simulink library "lib_controller"  (R2015a)
settings: Solver=ode45  StartTime=0.0  StopTime=10.0  RelTol=1e-3
values from neighbouring files (symbols this model uses):
  CG_0 = [0,0,0.02]'    [SetupComplete.m]
  g = 9.81    [SetupComplete.m]
  h_M = 0.064    [SetupComplete.m]
  I_BAC_0 = [ Ix,0,Ixz;0,Iy,0;Ixz,0,Iz]    [SetupComplete.m]
  l = 0.3450    (= 0.345)    [NDI_components.m]    (also in SetupComplete.m; robust_controller.m)
  m = 3.51    [SetupComplete.m]
  m_0 = 2.61    [SetupComplete.m]
  m_M = 0.300    (= 0.3)    [SetupComplete.m]
  T_sim = 0.01    [Run3Copter.m]
undefined symbols (not defined in the file or in its folder): Theta_1_roll_last, Theta_2_roll_last, Theta_3_roll_last, V_long_lastA_w_z, V_long_lastAoA, V_roll_last, V_yaw_last, W_long_lastA_w_z, W_long_lastAoA, W_roll_last, W_yaw_last
libraries: simulink x65, Adaptive_FaultTolerantControl x8, lib_controller x5, qcatlib x4, dspinverses x4, aerolibtransform2 x3, aerolib6dofsys x1
(part 9 of 10)

== matlab function lib_controller/Controller/NDI+CA Controller/4DOF NDI+CA Controller/F(X) ==
  data: fx output; prev_input input
function fx = fx(prev_input)
    % Calculates f_hat(x). The expression is calculated in NDI_components
    % x_dot = f(x) + g(x,u)
    %   g(x,u) ~= g(x,u0) + jac(g(x,u), u)(u0) * (u - u0)
    %   g(x,u) ~= h(x,u0) + jac(g(x,u), u)(u0) * u
    % x_dot = f_hat(x) + jac(g(x,u), u) * u
    %   f_hat(x) = f(x) + g(x,u0) - jac(g(x,u), u)(u0) *  u0
    %   g_hat(x) = jac(g(x,u), u)(u0)
    % x_dot = f_hat(x) + g_hat(x) * u
    Ixx = I_BAC(1,1);
    Iyy = I_BAC(2,2);
    Izz = I_BAC(3,3);
    Ixz = I_BAC(1,3);
    Iyz = I_BAC(2,3);
    cx = CG(1);
    cy = CG(2);
    cz = CG(3);
    tau1_0 = prev_input(1);
    eta1_0 = prev_input(2);
    gamma1_0 = prev_input(3);
    tau2_0 = prev_input(4);
    eta2_0 = prev_input(5);
    gamma2_0 = prev_input(6);
    tau3_0 = prev_input(7);
    eta3_0 = prev_input(8);
    gamma3_0 = prev_input(9);

    % TODO Precompute sines and cosines to improve performance. Some
    % repeated terms can also be precomputed
 fx = [...
               (88.941*(6.6073e-7*mass*P^2 + 0.000032054*mass*P*R - 6.6073e-7*mass*R^2 + 0.011243*V*mass*R + 0.011243*Gx - 0.011243*Q*W*mass - 5.7814e-6*eta1_0*mass*tau1_0*cos(eta1_0)))/mass;
 (88.941*(0.011243*Gy - 0.16865*eta1_0*tau1_0*cos(eta1_0) + 7.3537e-7*P*Q*mass + 0.00003163*Q*R*mass + 0.011243*P*W*mass - 0.011243*R*U*mass - 1.7153e-7*eta1_0*mass*tau1_0*sin(eta1_0)))/mass;
                                        -(88.941*(0.000016865*mass*P^2 + 0.011243*V*mass*P + 0.000016865*mass*Q^2 - 0.011243*U*mass*Q - 0.011243*Gz + 0.16865*eta1_0*tau1_0*sin(eta1_0)))/mass;
                                                                                                                               0.010171*eta1_0*tau1_0*sin(eta1_0) - 0.87546*Q*R - 0.043603*P*Q;
                                                                                                                  0.039177*P^2 + 0.90059*P*R - 0.039177*R^2 - 0.3428*eta1_0*tau1_0*cos(eta1_0);
                                                                                                                                0.043603*Q*R - 0.12686*P*Q - 0.20367*eta1_0*tau1_0*sin(eta1_0)];

== matlab function lib_controller/Controller/NDI+CA Controller/4DOF ANN+NDI+CA Controller - No massic update/Rotational Kinematics ==
  data: PQR output size=3; Eulerdot input size=3; Euler input size=3
function PQR = rot_kin(Eulerdot,Euler)
%solves rotational kinematic equations
Phi = Euler(1);
Theta = Euler(2);
Psi = Euler(3);
A = [1 sin(Phi)*tan(Theta) cos(Phi)*tan(Theta);
     0 cos(Phi) -sin(Phi);
     0 sin(Phi)*sec(Theta) cos(Phi)*sec(Theta)];
PQR = A'*Eulerdot;
end

== matlab function lib_controller/Controller/NDI+CA Controller/ 9DOF NDI+CA Controller - No massic update/F(X) 9DOF_UVWPQR ==
  data: fx output size=[6,1]; prev_input input size=[9,1]; gforce_body input size=[3,1]; omega_body input size=[3,1]; v_body input size=[3,1]
function fx = fx(prev_input, gforce_body, omega_body, v_body)
    % Calculates f_hat(x). The expression is calculated in NDI_components
    % x_dot = f(x) + g(x,u)
    %   g(x,u) ~= g(x,u0) + jac(g(x,u), u)(u0) * (u - u0)
    %   g(x,u) ~= h(x,u0) + jac(g(x,u), u)(u0) * u
    % x_dot = f_hat(x) + jac(g(x,u), u) * u
    %   f_hat(x) = f(x) + g(x,u0) - jac(g(x,u), u)(u0) *  u0
    %   g_hat(x) = jac(g(x,u), u)(u0)
    % x_dot = f_hat(x) + g_hat(x) * u
    tau1_0 = prev_input(1);
    eta1_0 = prev_input(2);
    gamma1_0 = prev_input(3);
    tau2_0 = prev_input(4);
    eta2_0 = prev_input(5);
    gamma2_0 = prev_input(6);
    tau3_0 = prev_input(7);
    eta3_0 = prev_input(8);
    gamma3_0 = prev_input(9);
    Gx =  gforce_body(1);
    Gy =  gforce_body(2);
    Gz =  gforce_body(3);
    U = v_body(1);
    V = v_body(2);
    W = v_body(3);
    P = omega_body(1);
    Q = omega_body(2);
    R = omega_body(3);

    % This matrix was precomputed in NDI_components.m
    % TODO Precompute sines and cosines to improve performance. Some
    % repeated terms can also be precomputed
    
 fx = [...
 5.88e-5*P^2 + 0.00285*P*R - 5.88e-5*R^2 + 1.0*V*R + 0.285*Gx - 1.0*Q*W + 4.27*gamma1_0*tau1_0*cos(gamma1_0) + 5.14e-4*gamma2_0*tau2_0*cos(gamma2_0) + 5.14e-4*gamma3_0*tau3_0*cos(gamma3_0) - 5.14e-4*eta1_0*tau1_0*cos(eta1_0)*cos(gamma1_0) + 4.27*eta2_0*tau2_0*cos(eta2_0)*cos(gamma2_0) + 4.27*eta3_0*tau3_0*cos(eta3_0)*cos(gamma3_0) + 0.038*eta1_0*tau1_0*cos(gamma1_0)*sin(eta1_0) - 0.019*eta2_0*tau2_0*cos(gamma2_0)*sin(eta2_0) - 0.019*eta3_0*tau3_0*cos(gamma3_0)*sin(eta3_0) + 0.038*gamma1_0*tau1_0*cos(eta1_0)*sin(gamma1_0) - 0.019*gamma2_0*tau2_0*cos(eta2_0)*sin(gamma2_0) - 0.019*gamma3_0*tau3_0*cos(eta3_0)*sin(gamma3_0) + 5.14e-4*gamma1_0*tau1_0*sin(eta1_0)*sin(gamma1_0) - 4.27*gamma2_0*tau2_0*sin(eta2_0)*sin(gamma2_0) - 4.27*gamma3_0*tau3_0*sin(eta3_0)*sin(gamma3_0);
        0.285*Gy + 6.54e-5*P*Q + 0.00281*Q*R + 1.0*P*W - 1.0*R*U - 6.56e-4*gamma1_0*tau1_0*cos(gamma1_0) - 4.27*gamma2_0*tau2_0*cos(gamma2_0) - 4.27*gamma3_0*tau3_0*cos(gamma3_0) - 4.27*eta1_0*tau1_0*cos(eta1_0)*cos(gamma1_0) - 3.21e-4*eta2_0*tau2_0*cos(eta2_0)*cos(gamma2_0) + 0.00163*eta3_0*tau3_0*cos(eta3_0)*cos(gamma3_0) - 1.53e-5*eta1_0*tau1_0*cos(gamma1_0)*sin(eta1_0) + 0.042*eta2_0*tau2_0*cos(gamma2_0)*sin(eta2_0) - 0.042*eta3_0*tau3_0*cos(gamma3_0)*sin(eta3_0) - 1.53e-5*gamma1_0*tau1_0*cos(eta1_0)*sin(gamma1_0) + 0.042*gamma2_0*tau2_0*cos(eta2_0)*sin(gamma2_0) - 0.042*gamma3_0*tau3_0*cos(eta3_0)*sin(gamma3_0) + 4.27*gamma1_0*tau1_0*sin(eta1_0)*sin(gamma1_0) + 3.21e-4*gamma2_0*tau2_0*sin(eta2_0)*sin(gamma2_0) - 0.00163*gamma3_0*tau3_0*sin(eta3_0)*sin(gamma3_0);
                                                                                                                                                                                                                                                                                                                                                                                                                                                - 0.0015*P^2 - 1.0*V*P - 0.0015*Q^2 + 1.0*U*Q + 0.285*Gz - 4.27*eta1_0*tau1_0*cos(gamma1_0)*sin(eta1_0) - 4.27*eta2_0*tau2_0*cos(gamma2_0)*sin(eta2_0) - 4.27*eta3_0*tau3_0*cos(gamma3_0)*sin(eta3_0) - 4.27*gamma1_0*tau1_0*cos(eta1_0)*sin(gamma1_0) - 4.27*gamma2_0*tau2_0*cos(eta2_0)*sin(gamma2_0) - 4.27*gamma3_0*tau3_0*cos(eta3_0)*sin(gamma3_0);
                                                        0.437*gamma1_0*tau1_0*cos(gamma1_0) - 0.876*Q*R - 0.0436*P*Q - 0.235*gamma2_0*tau2_0*cos(gamma2_0) - 0.235*gamma3_0*tau3_0*cos(gamma3_0) + 0.893*eta1_0*tau1_0*cos(eta1_0)*cos(gamma1_0) + 0.214*eta2_0*tau2_0*cos(eta2_0)*cos(gamma2_0) - 1.09*eta3_0*tau3_0*cos(eta3_0)*cos(gamma3_0) + 0.0102*eta1_0*tau1_0*cos(gamma1_0)*sin(eta1_0) - 28.0*eta2_0*tau2_0*cos(gamma2_0)*sin(eta2_0) + 28.0*eta3_0*tau3_0*cos(gamma3_0)*sin(eta3_0) + 0.0102*gamma1_0*tau1_0*cos(eta1_0)*sin(gamma1_0) - 28.0*gamma2_0*tau2_0*cos(eta2_0)*sin(gamma2_0) + 28.0*gamma3_0*tau3_0*cos(eta3_0)*sin(gamma3_0) - 0.893*gamma1_0*tau1_0*sin(eta1_0)*sin(gamma1_0) - 0.214*gamma2_0*tau2_0*sin(eta2_0)*sin(gamma2_0) + 1.09*gamma3_0*tau3_0*sin(eta3_0)*sin(gamma3_0);
                                                  0.0392*P^2 + 0.901*P*R - 0.0392*R^2 + 0.11*gamma1_0*tau1_0*cos(gamma1_0) + 0.343*gamma2_0*tau2_0*cos(gamma2_0) + 0.343*gamma3_0*tau3_0*cos(gamma3_0) - 0.343*eta1_0*tau1_0*cos(eta1_0)*cos(gamma1_0) + 0.11*eta2_0*tau2_0*cos(eta2_0)*cos(gamma2_0) + 0.11*eta3_0*tau3_0*cos(eta3_0)*cos(gamma3_0) + 25.3*eta1_0*tau1_0*cos(gamma1_0)*sin(eta1_0) - 12.7*eta2_0*tau2_0*cos(gamma2_0)*sin(eta2_0) - 12.7*eta3_0*tau3_0*cos(gamma3_0)*sin(eta3_0) + 25.3*gamma1_0*tau1_0*cos(eta1_0)*sin(gamma1_0) - 12.7*gamma2_0*tau2_0*cos(eta2_0)*sin(gamma2_0) - 12.7*gamma3_0*tau3_0*cos(eta3_0)*sin(gamma3_0) + 0.343*gamma1_0*tau1_0*sin(eta1_0)*sin(gamma1_0) - 0.11*gamma2_0*tau2_0*sin(eta2_0)*sin(gamma2_0) - 0.11*gamma3_0*tau3_0*sin(eta3_0)*sin(gamma3_0);
                                                           0.0436*Q*R - 0.127*P*Q - 0.0102*gamma1_0*tau1_0*cos(gamma1_0) + 7.53*gamma2_0*tau2_0*cos(gamma2_0) + 7.53*gamma3_0*tau3_0*cos(gamma3_0) - 15.1*eta1_0*tau1_0*cos(eta1_0)*cos(gamma1_0) - 13.0*eta2_0*tau2_0*cos(eta2_0)*cos(gamma2_0) + 13.0*eta3_0*tau3_0*cos(eta3_0)*cos(gamma3_0) - 0.204*eta1_0*tau1_0*cos(gamma1_0)*sin(eta1_0) + 0.855*eta2_0*tau2_0*cos(gamma2_0)*sin(eta2_0) - 0.448*eta3_0*tau3_0*cos(gamma3_0)*sin(eta3_0) - 0.204*gamma1_0*tau1_0*cos(eta1_0)*sin(gamma1_0) + 0.855*gamma2_0*tau2_0*cos(eta2_0)*sin(gamma2_0) - 0.448*gamma3_0*tau3_0*cos(eta3_0)*sin(gamma3_0) + 15.1*gamma1_0*tau1_0*sin(eta1_0)*sin(gamma1_0) + 13.0*gamma2_0*tau2_0*sin(eta2_0)*sin(gamma2_0) - 13.0*gamma3_0*tau3_0*sin(eta3_0)*sin(gamma3_0)];

== matlab function lib_controller/Controller/NDI+CA Controller/ 9DOF NDI+CA Controller - No massic update/G(X) 9DOF_UVWPQR ==
  data: gx output size=[6,9]; prev_input input size=[9,1]
function gx = gx(prev_input)
    % Calculates f_hat(x). The expression is calculated in NDI_components
    % x_dot = f(x) + g(x,u)
    %   g(x,u) ~= g(x,u0) + jac(g(x,u), u)(u0) * (u - u0)
    %   g(x,u) ~= h(x,u0) + jac(g(x,u), u)(u0) * u
    % x_dot = f_hat(x) + jac(g(x,u), u) * u
    %   f_hat(x) = f(x) + g(x,u0) - jac(g(x,u), u)(u0) *  u0
    %   g_hat(x) = jac(g(x,u), u)(u0)
    % x_dot = f_hat(x) + g_hat(x) * u
    tau1_0 = prev_input(1);
    eta1_0 = prev_input(2);
    gamma1_0 = prev_input(3);
    tau2_0 = prev_input(4);
    eta2_0 = prev_input(5);
    gamma2_0 = prev_input(6);
    tau3_0 = prev_input(7);
    eta3_0 = prev_input(8);
    gamma3_0 = prev_input(9);
    
    % This matrix was precomputed in NDI_components.m
    % TODO Precompute sines and cosines to improve performance. Some
    % repeated terms can also be precomputed
    gx = [...
   5.14e-4*cos(gamma1_0)*sin(eta1_0) - 4.27*sin(gamma1_0) + 0.038*cos(eta1_0)*cos(gamma1_0),  5.14e-4*tau1_0*cos(eta1_0)*cos(gamma1_0) - 0.038*tau1_0*cos(gamma1_0)*sin(eta1_0), - 4.27*tau1_0*cos(gamma1_0) - 0.038*tau1_0*cos(eta1_0)*sin(gamma1_0) - 5.14e-4*tau1_0*sin(eta1_0)*sin(gamma1_0), - 5.14e-4*sin(gamma2_0) - 4.27*cos(gamma2_0)*sin(eta2_0) - 0.019*cos(eta2_0)*cos(gamma2_0),    0.019*tau2_0*cos(gamma2_0)*sin(eta2_0) - 4.27*tau2_0*cos(eta2_0)*cos(gamma2_0), 0.019*tau2_0*cos(eta2_0)*sin(gamma2_0) - 5.14e-4*tau2_0*cos(gamma2_0) + 4.27*tau2_0*sin(eta2_0)*sin(gamma2_0), - 5.14e-4*sin(gamma3_0) - 4.27*cos(gamma3_0)*sin(eta3_0) - 0.019*cos(eta3_0)*cos(gamma3_0),    0.019*tau3_0*cos(gamma3_0)*sin(eta3_0) - 4.27*tau3_0*cos(eta3_0)*cos(gamma3_0), 0.019*tau3_0*cos(eta3_0)*sin(gamma3_0) - 5.14e-4*tau3_0*cos(gamma3_0) + 4.27*tau3_0*sin(eta3_0)*sin(gamma3_0);
 6.56e-4*sin(gamma1_0) + 4.27*cos(gamma1_0)*sin(eta1_0) - 1.53e-5*cos(eta1_0)*cos(gamma1_0),   4.27*tau1_0*cos(eta1_0)*cos(gamma1_0) + 1.53e-5*tau1_0*cos(gamma1_0)*sin(eta1_0), 6.56e-4*tau1_0*cos(gamma1_0) + 1.53e-5*tau1_0*cos(eta1_0)*sin(gamma1_0) - 4.27*tau1_0*sin(eta1_0)*sin(gamma1_0),   4.27*sin(gamma2_0) + 3.21e-4*cos(gamma2_0)*sin(eta2_0) + 0.042*cos(eta2_0)*cos(gamma2_0), 3.21e-4*tau2_0*cos(eta2_0)*cos(gamma2_0) - 0.042*tau2_0*cos(gamma2_0)*sin(eta2_0), 4.27*tau2_0*cos(gamma2_0) - 0.042*tau2_0*cos(eta2_0)*sin(gamma2_0) - 3.21e-4*tau2_0*sin(eta2_0)*sin(gamma2_0),   4.27*sin(gamma3_0) - 0.00163*cos(gamma3_0)*sin(eta3_0) - 0.042*cos(eta3_0)*cos(gamma3_0), 0.042*tau3_0*cos(gamma3_0)*sin(eta3_0) - 0.00163*tau3_0*cos(eta3_0)*cos(gamma3_0), 4.27*tau3_0*cos(gamma3_0) + 0.042*tau3_0*cos(eta3_0)*sin(gamma3_0) + 0.00163*tau3_0*sin(eta3_0)*sin(gamma3_0);
                                                            -4.27*cos(eta1_0)*cos(gamma1_0),                                              4.27*tau1_0*cos(gamma1_0)*sin(eta1_0),                                                                           4.27*tau1_0*cos(eta1_0)*sin(gamma1_0),                                                            -4.27*cos(eta2_0)*cos(gamma2_0),                                             4.27*tau2_0*cos(gamma2_0)*sin(eta2_0),                                                                         4.27*tau2_0*cos(eta2_0)*sin(gamma2_0),                                                            -4.27*cos(eta3_0)*cos(gamma3_0),                                             4.27*tau3_0*cos(gamma3_0)*sin(eta3_0),                                                                         4.27*tau3_0*cos(eta3_0)*sin(gamma3_0);
   0.0102*cos(eta1_0)*cos(gamma1_0) - 0.893*cos(gamma1_0)*sin(eta1_0) - 0.437*sin(gamma1_0), - 0.893*tau1_0*cos(eta1_0)*cos(gamma1_0) - 0.0102*tau1_0*cos(gamma1_0)*sin(eta1_0),   0.893*tau1_0*sin(eta1_0)*sin(gamma1_0) - 0.0102*tau1_0*cos(eta1_0)*sin(gamma1_0) - 0.437*tau1_0*cos(gamma1_0),     0.235*sin(gamma2_0) - 0.214*cos(gamma2_0)*sin(eta2_0) - 28.0*cos(eta2_0)*cos(gamma2_0),    28.0*tau2_0*cos(gamma2_0)*sin(eta2_0) - 0.214*tau2_0*cos(eta2_0)*cos(gamma2_0),   0.235*tau2_0*cos(gamma2_0) + 28.0*tau2_0*cos(eta2_0)*sin(gamma2_0) + 0.214*tau2_0*sin(eta2_0)*sin(gamma2_0),      0.235*sin(gamma3_0) + 1.09*cos(gamma3_0)*sin(eta3_0) + 28.0*cos(eta3_0)*cos(gamma3_0),     1.09*tau3_0*cos(eta3_0)*cos(gamma3_0) - 28.0*tau3_0*cos(gamma3_0)*sin(eta3_0),    0.235*tau3_0*cos(gamma3_0) - 28.0*tau3_0*cos(eta3_0)*sin(gamma3_0) - 1.09*tau3_0*sin(eta3_0)*sin(gamma3_0);
      0.343*cos(gamma1_0)*sin(eta1_0) - 0.11*sin(gamma1_0) + 25.3*cos(eta1_0)*cos(gamma1_0),     0.343*tau1_0*cos(eta1_0)*cos(gamma1_0) - 25.3*tau1_0*cos(gamma1_0)*sin(eta1_0),    - 0.11*tau1_0*cos(gamma1_0) - 25.3*tau1_0*cos(eta1_0)*sin(gamma1_0) - 0.343*tau1_0*sin(eta1_0)*sin(gamma1_0),    - 0.343*sin(gamma2_0) - 0.11*cos(gamma2_0)*sin(eta2_0) - 12.7*cos(eta2_0)*cos(gamma2_0),     12.7*tau2_0*cos(gamma2_0)*sin(eta2_0) - 0.11*tau2_0*cos(eta2_0)*cos(gamma2_0),    12.7*tau2_0*cos(eta2_0)*sin(gamma2_0) - 0.343*tau2_0*cos(gamma2_0) + 0.11*tau2_0*sin(eta2_0)*sin(gamma2_0),    - 0.343*sin(gamma3_0) - 0.11*cos(gamma3_0)*sin(eta3_0) - 12.7*cos(eta3_0)*cos(gamma3_0),     12.7*tau3_0*cos(gamma3_0)*sin(eta3_0) - 0.11*tau3_0*cos(eta3_0)*cos(gamma3_0),    12.7*tau3_0*cos(eta3_0)*sin(gamma3_0) - 0.343*tau3_0*cos(gamma3_0) + 0.11*tau3_0*sin(eta3_0)*sin(gamma3_0);
    0.0102*sin(gamma1_0) + 15.1*cos(gamma1_0)*sin(eta1_0) - 0.204*cos(eta1_0)*cos(gamma1_0),     15.1*tau1_0*cos(eta1_0)*cos(gamma1_0) + 0.204*tau1_0*cos(gamma1_0)*sin(eta1_0),    0.0102*tau1_0*cos(gamma1_0) + 0.204*tau1_0*cos(eta1_0)*sin(gamma1_0) - 15.1*tau1_0*sin(eta1_0)*sin(gamma1_0),      13.0*cos(gamma2_0)*sin(eta2_0) - 7.53*sin(gamma2_0) + 0.855*cos(eta2_0)*cos(gamma2_0),    13.0*tau2_0*cos(eta2_0)*cos(gamma2_0) - 0.855*tau2_0*cos(gamma2_0)*sin(eta2_0),  - 7.53*tau2_0*cos(gamma2_0) - 0.855*tau2_0*cos(eta2_0)*sin(gamma2_0) - 13.0*tau2_0*sin(eta2_0)*sin(gamma2_0),    - 7.53*sin(gamma3_0) - 13.0*cos(gamma3_0)*sin(eta3_0) - 0.448*cos(eta3_0)*cos(gamma3_0),    0.448*tau3_0*cos(gamma3_0)*sin(eta3_0) - 13.0*tau3_0*cos(eta3_0)*cos(gamma3_0),    0.448*tau3_0*cos(eta3_0)*sin(gamma3_0) - 7.53*tau3_0*cos(gamma3_0) + 13.0*tau3_0*sin(eta3_0)*sin(gamma3_0)];
 
    
    
    
    
%  0.038016*cos(eta1_0) + 0.00051422*sin(eta1_0), 0.00051422*tau1_0*cos(eta1_0) - 0.038016*tau1_0*sin(eta1_0),    -4.2737*tau1_0, -0.019008,    -4.2737*tau2_0, -0.00051422*tau2_0, -0.019008,   -4.2737*tau3_0, -0.00051422*tau3_0;
%   4.2748*sin(eta1_0) - 0.000015257*cos(eta1_0),  4.2748*tau1_0*cos(eta1_0) + 0.000015257*tau1_0*sin(eta1_0), 0.00065622*tau1_0,  0.042029, 0.00032056*tau2_0,      4.2732*tau2_0, -0.041999, -0.001633*tau3_0,      4.2732*tau3_0;
%                            -4.2735*cos(eta1_0),                                   4.2735*tau1_0*sin(eta1_0),                 0,   -4.2735,                 0,                  0,   -4.2735,                0,                  0;
%     0.010171*cos(eta1_0) - 0.89255*sin(eta1_0),  - 0.89255*tau1_0*cos(eta1_0) - 0.010171*tau1_0*sin(eta1_0),   -0.43748*tau1_0,    -28.02,   -0.21371*tau2_0,     0.23535*tau2_0,    27.999,    1.0887*tau3_0,     0.23535*tau3_0;
%       25.344*cos(eta1_0) + 0.34281*sin(eta1_0),      0.34281*tau1_0*cos(eta1_0) - 25.344*tau1_0*sin(eta1_0),   -0.11019*tau1_0,   -12.672,   -0.11019*tau2_0,    -0.34281*tau2_0,   -12.672,  -0.11019*tau3_0,    -0.34281*tau3_0;
%        15.06*sin(eta1_0) - 0.20367*cos(eta1_0),       15.06*tau1_0*cos(eta1_0) + 0.20367*tau1_0*sin(eta1_0),   0.010171*tau1_0,   0.85486,     13.029*tau2_0,     -7.5251*tau2_0,  -0.44753,    -13.05*tau3_0,     -7.5251*tau3_0];

== matlab function lib_controller/Controller/NDI+CA Controller/4DOF ANN+NDI+CA Controller - No massic update/G(X) 4DOF_WPQR ==
  data: gx output size=[4,4]; prev_input input size=[9,1]
function gx = gx(prev_input)
    % Calculates f_hat(x). The expression is calculated in NDI_components
    % x_dot = f(x) + g(x,u)
    %   g(x,u) ~= g(x,u0) + jac(g(x,u), u)(u0) * (u - u0)
    %   g(x,u) ~= h(x,u0) + jac(g(x,u), u)(u0) * u
    % x_dot = f_hat(x) + jac(g(x,u), u) * u
    %   f_hat(x) = f(x) + g(x,u0) - jac(g(x,u), u)(u0) *  u0
    %   g_hat(x) = jac(g(x,u), u)(u0)
    % x_dot = f_hat(x) + g_hat(x) * u
    tau1_0 = prev_input(1);
    eta1_0 = prev_input(2);
    gamma1_0 = prev_input(3);
    tau2_0 = prev_input(4);
    eta2_0 = prev_input(5);
    gamma2_0 = prev_input(6);
    tau3_0 = prev_input(7);
    eta3_0 = prev_input(8);
    gamma3_0 = prev_input(9);
    
    % This matrix was precomputed in NDI_components.m
    % TODO Precompute sines and cosines to improve performance. Some
    % repeated terms can also be precomputed
    
    % Kt = 29.6 Kq = 0.3
    gx = [...
                          -7.379*cos(eta1_0),                                7.379*tau1_0*sin(eta1_0), -7.379,  -7.379;
     0.04359*cos(eta1_0) - 1.541*sin(eta1_0), - 1.541*tau1_0*cos(eta1_0) - 0.04359*tau1_0*sin(eta1_0), -48.41,   48.32;
       43.76*cos(eta1_0) + 1.469*sin(eta1_0),     1.469*tau1_0*cos(eta1_0) - 43.76*tau1_0*sin(eta1_0), -21.88,  -21.88;
       26.0*sin(eta1_0) - 0.8729*cos(eta1_0),     26.0*tau1_0*cos(eta1_0) + 0.8729*tau1_0*sin(eta1_0),  1.997, -0.2515];
 
% Kt = 15 Kq = 0.07
%                        -4.274*cos(eta1_0),                                 4.274*tau1_0*sin(eta1_0), -4.274,  -4.274;
%  0.01017*cos(eta1_0) - 0.8926*sin(eta1_0), - 0.8926*tau1_0*cos(eta1_0) - 0.01017*tau1_0*sin(eta1_0), -28.02,    28.0;
%    25.34*cos(eta1_0) + 0.3428*sin(eta1_0),     0.3428*tau1_0*cos(eta1_0) - 25.34*tau1_0*sin(eta1_0), -12.67,  -12.67;
%    15.06*sin(eta1_0) - 0.2037*cos(eta1_0),     15.06*tau1_0*cos(eta1_0) + 0.2037*tau1_0*sin(eta1_0), 0.8549, -0.4475];

== matlab function lib_controller/Controller/NDI+CA Controller/4DOF ANN+NDI+CA Controller - No massic update/Adaptive NN/Crossed NN/Cross NN ==
  data: X_bar input size=[30,1]; v_ad_comp output size=4; e input size=6; P input size=[6,6]; B input size=[6,4]; learning_rate input size=1; Reg_param input size=2; W input size=[4,51]; V input size=[50,30]; v_ad output size=4; Z_norm_unit output size=1; T_sim parameter size=1; W_update output size=[4,51]; V_update output size=[50,30]
function [v_ad_comp,v_ad,Z_norm_unit,W_update,V_update]  = Cross_NN(X_bar,e, P, B,learning_rate,Reg_param,W,V,T_sim)

%% Compute prelimiary parameters 
zeta= e'*P*B;

%% Feedforward
z = V*X_bar;
s=sigmoid(V*X_bar);

sigma = [1 ; s ];
% v_ad = W*sigma;

sigma_grad = (sigma.*(ones(size(sigma))-sigma));

%% Compute the gradients or adaptation laws
Gamma_w= learning_rate; % W learnign rate
Gamma_v= learning_rate; %V learning rate
lambda_v = Reg_param(1);
lambda_w = Reg_param(2);

V_dot=zeros(size(V));
W_dot=zeros(size(W));

W_dot= -Gamma_w*(  (sigma - sigma_grad.*[1;z] )*zeta  )';
W_dot(:,2:end)= W_dot(:,2:end) - Gamma_w*lambda_w*norm(zeta)*(W(:,2:end));

M = W'*zeta'.*sigma_grad ;
V_dot= -Gamma_v*( M(2:end)*X_bar'  );
V_dot(:,2:end)= V_dot(:,2:end) - Gamma_v*lambda_v*norm(zeta).*V(:,2:end);

% % % % Other way: Based on notes of Andrew NG
% % % 
% % % delta2=W'*zeta'.*sigma_grad;
% % % 
% % % V_dot = - Gamma_v*( delta2(2:end)*X_bar');
% % % V_dot(:,2:end)= V_dot(:,2:end) - Gamma_v*lambda*norm(zeta).*V(:,2:end);
% % % 
% % % W_dot = - Gamma_w*( sigma*zeta)';
% % % W_dot(:,2:end)= W_dot(:,2:end) - Gamma_w*lambda*norm(zeta)*(W(:,2:end));

%% Adaptation scalled with loop time
W_update = W + T_sim*W_dot;
V_update = V + T_sim*V_dot;

%% Re-compute v_ad
s=sigmoid(V_update*X_bar);

sigma = [1 ; s(:,1) ];
v_ad = W_update*sigma;

%% Compute v_ad_comp (add robustifying terms)
Z = [ V,zeros(size(V,1),size(W,2));
    zeros(size(W,1),size(V,2)),W];
    
Z_norm = norm(Z,'fro');
% Z_max = 2*min(size(W,1),size(W,2) )*min(size(V,1),size(V,2));
Z_max = 1;
Z_norm_unit = Z_norm;

% K_r0= 0.02;
% K_r1= 0;
K_r0= 1;
K_r1= 1;

v_r0 = -K_r0*zeta';
v_r1 = -K_r1*(Z_norm+Z_max)*zeta';

v_ad_comp = v_ad + v_r1 +v_r0;
end

== matlab function lib_controller/Controller/NDI+CA Controller/4DOF ANN+NDI+CA Controller - No massic update/Rotational Kinematics1 ==
  data: PQR input size=3; Eulerdot output size=3; Euler input size=3
function Eulerdot = rot_kin(PQR,Euler)
%solves rotational kinematic equations
Phi = Euler(1);
Theta = Euler(2);
Psi = Euler(3);
A = [1 sin(Phi)*tan(Theta) cos(Phi)*tan(Theta);
     0 cos(Phi) -sin(Phi);
     0 sin(Phi)*sec(Theta) cos(Phi)*sec(Theta)];
Eulerdot = A*PQR;
end

== matlab function lib_controller/Controller/NDI+CA Controller/4DOF ANN+NDI+CA Controller - No massic update/Sigmoid /MATLAB Function ==
  data: u input; y output; a input
function y = sigmoid_a(u,a)

y = 2.0 ./ (1.0 + exp(-a*u(:)))-1;

== matlab function lib_controller/Controller/NDI+CA Controller/4DOF ANN+NDI+CA Controller - No massic update/F(X) ==
  data: fx output size=[4,1]; prev_input input size=[9,1]; gforce_body input size=[3,1]; omega_body input size=[3,1]; v_body input size=[3,1]
function fx = fx(prev_input, gforce_body, omega_body, v_body)
    % Calculates f_hat(x). The expression is calculated in NDI_components
    % x_dot = f(x) + g(x,u)
    %   g(x,u) ~= g(x,u0) + jac(g(x,u), u)(u0) * (u - u0)
    %   g(x,u) ~= h(x,u0) + jac(g(x,u), u)(u0) * u
    % x_dot = f_hat(x) + jac(g(x,u), u) * u
    %   f_hat(x) = f(x) + g(x,u0) - jac(g(x,u), u)(u0) *  u0
    %   g_hat(x) = jac(g(x,u), u)(u0)
    % x_dot = f_hat(x) + g_hat(x) * u
    tau1_0 = prev_input(1);
    eta1_0 = prev_input(2);
    gamma1_0 = prev_input(3);
    tau2_0 = prev_input(4);
    eta2_0 = prev_input(5);
    gamma2_0 = prev_input(6);
    tau3_0 = prev_input(7);
    eta3_0 = prev_input(8);
    gamma3_0 = prev_input(9);
    Gx =  gforce_body(1);
    Gy =  gforce_body(2);
    Gz =  gforce_body(3);
    U = v_body(1);
    V = v_body(2);
    W = v_body(3);
    P = omega_body(1);
    Q = omega_body(2);
    R = omega_body(3);

    % This matrix was precomputed in NDI_components.m
    % TODO Precompute sines and cosines to improve performance. Some
    % repeated terms can also be precomputed
    
 % Kt = 29.6 Kq = 0.3
 fx = [... 
                    - 0.0015*P^2 - 1.0*V*P - 0.0015*Q^2 + U*Q + 0.2849*Gz - 7.379*eta1_0*tau1_0*sin(eta1_0);
              1.541*eta1_0*tau1_0*cos(eta1_0) - 0.8756*Q*R - 0.0436*P*Q + 0.04359*eta1_0*tau1_0*sin(eta1_0);
 0.03918*P^2 + 0.9007*P*R - 0.03918*R^2 - 1.469*eta1_0*tau1_0*cos(eta1_0) + 43.76*eta1_0*tau1_0*sin(eta1_0);
                0.0436*Q*R - 0.1269*P*Q - 26.0*eta1_0*tau1_0*cos(eta1_0) - 0.8729*eta1_0*tau1_0*sin(eta1_0)];    
 
% Kt = 15 Kq = 0.07
%                          - 0.0015*P^2 - 1.0*V*P - 0.0015*Q^2 + 1.0*U*Q + 0.2849*Gz - 4.2735*eta1_0*tau1_0*sin(eta1_0);
%                   0.89255*eta1_0*tau1_0*cos(eta1_0) - 0.87555*Q*R - 0.043605*P*Q + 0.010171*eta1_0*tau1_0*sin(eta1_0);
%      0.039179*P^2 + 0.90066*P*R - 0.039179*R^2 - 0.34281*eta1_0*tau1_0*cos(eta1_0) + 25.344*eta1_0*tau1_0*sin(eta1_0);
%                      0.043605*Q*R - 0.12686*P*Q - 15.06*eta1_0*tau1_0*cos(eta1_0) - 0.20367*eta1_0*tau1_0*sin(eta1_0)];

== matlab function lib_controller/Controller/NDI+CA Controller/4DOF ANN+NDI+CA Controller - No massic update/Rotational Kinematics2 ==
  data: PQR output size=3; Eulerdot input size=3; Euler input size=3
function PQR = rot_kin(Eulerdot,Euler)
%solves rotational kinematic equations
Phi = Euler(1);
Theta = Euler(2);
Psi = Euler(3);
A = [1 sin(Phi)*tan(Theta) cos(Phi)*tan(Theta);
     0 cos(Phi) -sin(Phi);
     0 sin(Phi)*sec(Theta) cos(Phi)*sec(Theta)];
PQR = A'*Eulerdot;
end

== matlab function lib_controller/Controller/NDI+CA Controller/4DOF ANN+NDI+CA Controller - No massic update/On-line (adaptive) multi-layer NNs/Pitch Channel/Long HL NN A_w_z/Long NN ==
  data: X_bar input size=[10,1]; v_ad_comp output; e input; F input; Ks input; B input; Long_learnign_rate input size=1; Long_reg_param input size=1; W input size=[1,31]; V input size=[30,10]; v_ad output; Z_norm_unit output; T_sim parameter; W_update output; V_update output
function [v_ad_comp,v_ad,Z_norm_unit,W_update,V_update]  = Long_AoA_NN(X_bar,e, F, Ks,B,Long_learnign_rate,Long_reg_param,W,V,T_sim)

%% Compute prelimiary parametes Ks(1)=K_b_alpha  and Ks(2) = K_b_q
P = [   1/Ks(1) , F/(Ks(1)^2+Ks(1)*Ks(2));
     1/(Ks(1)^2+Ks(1)*Ks(2)) ,(Ks(1)^2+Ks(1)*Ks(2)+F^2)/(Ks(2)^2*Ks(1)+Ks(2)*Ks(1)^2) ];
zeta= e'*P*B;
s=zeros(30,1);
z=s;
%% Feedforward
z = V*X_bar;
s=sigmoid(V*X_bar);

sigma = [1 ; s ];
% v_ad = W*sigma;

sigma_grad = (sigma.*(ones(size(sigma))-sigma));

%% Compute the gradients or adaptation laws
Gamma_w= Long_learnign_rate; % W learnign rate
Gamma_v= Long_learnign_rate; %V learning rate
lambda = Long_reg_param;

V_dot=zeros(size(V));
W_dot=zeros(size(W'));

W_dot= -Gamma_w*(  (sigma - sigma_grad.*[1;z] ).*zeta  );
W_dot(2:end,1)= W_dot(2:end,1) - Gamma_w*lambda*norm(zeta)*(W(:,2:end))';

M = W'*zeta.*sigma_grad ;
V_dot= -Gamma_v*( M(2:end)*X_bar'  );
V_dot(:,2:end)= V_dot(:,2:end) - Gamma_v*lambda*norm(zeta).*V(:,2:end);


% % % Other way: Based on notes of Andrew NG
% % W_dot=zeros(size(W));
% % delta2=W'*zeta.*sigma_grad;
% % 
% % V_dot = - Gamma_v*( delta2(2:end)*X_bar');
% % V_dot(:,2:end)= V_dot(:,2:end) - Gamma_v*lambda*norm(zeta).*V(:,2:end);
% % 
% % W_dot = - Gamma_w*( zeta*sigma');
% % W_dot(:,2:end)= W_dot(:,2:end) - Gamma_w*lambda*norm(zeta)*(W(:,2:end));
% % 
% % W_dot = W_dot';


%% Adaptation
W_update = W + T_sim*W_dot';
V_update = V + T_sim*V_dot;

%% re-compute v_ad

z = V*X_bar;
s=sigmoid(V*X_bar);

sigma = [1 ; s(:,1) ];
v_ad = W*sigma;

%% Compute v_ad_comp
Z = [ V,zeros(size(V,1),size(W,2));
    zeros(size(W,1),size(V,2)),W];
    
Z_norm = norm(Z,'fro');
Z_max = 2*min(size(W,1),size(W,2) )*min( size(V,1),size(V,2) );
Z_norm_unit = Z_norm/Z_max;

K_r0= 0.1;
K_r1= 0.001;
v_r0 = -K_r0*zeta;
v_r1 = -K_r1*(Z_norm+Z_max)*zeta;

v_ad_comp = v_ad + v_r1 +v_r0;


end

== matlab function lib_controller/Controller/NDI+CA Controller/4DOF ANN+NDI+CA Controller - No massic update/On-line (adaptive) multi-layer NNs/Pitch Channel/Long HL NN AoA/Long NN ==
  data: X_bar input size=[10,1]; v_ad_comp output; e input; Ks input; B input; Long_learnign_rate input size=1; Long_reg_param input size=1; W input size=[1,31]; V input size=[30,10]; v_ad output; Z_norm_unit output; T_sim parameter; W_update output; V_update output
function [v_ad_comp,v_ad,Z_norm_unit,W_update,V_update]  = Long_AoA_NN(X_bar,e, Ks,B,Long_learnign_rate,Long_reg_param,W,V,T_sim)

%% Compute prelimiary parametes Ks(1)=K_b_alpha  and Ks(2) = K_b_q
P = [   1/Ks(1) , 1/(Ks(1)^2+Ks(1)*Ks(2));
     1/(Ks(1)^2+Ks(1)*Ks(2)) ,(Ks(1)^2+Ks(1)*Ks(2)+1)/(Ks(2)^2*Ks(1)+Ks(2)*Ks(1)^2) ];
zeta= e'*P*B;
s=zeros(30,1);
z=s;
%% Feedforward
z = V*X_bar;
s=sigmoid(V*X_bar);

sigma = [1 ; s ];
% v_ad = W*sigma;

sigma_grad = (sigma.*(ones(size(sigma))-sigma));

%% Compute the gradients or adaptation laws
Gamma_w= Long_learnign_rate; % W learnign rate
Gamma_v= Long_learnign_rate; %V learning rate
lambda = Long_reg_param;

V_dot=zeros(size(V));
W_dot=zeros(size(W'));

W_dot= -Gamma_w*(  (sigma - sigma_grad.*[1;z] ).*zeta  );
W_dot(2:end,1)= W_dot(2:end,1) - Gamma_w*lambda*norm(zeta)*(W(:,2:end))';

M = W'*zeta.*sigma_grad ;
V_dot= -Gamma_v*( M(2:end)*X_bar'  );
V_dot(:,2:end)= V_dot(:,2:end) - Gamma_v*lambda*norm(zeta).*V(:,2:end);


% % % Other way: Based on notes of Andrew NG
% % W_dot=zeros(size(W));
% % delta2=W'*zeta.*sigma_grad;
% % 
% % V_dot = - Gamma_v*( delta2(2:end)*X_bar');
% % V_dot(:,2:end)= V_dot(:,2:end) - Gamma_v*lambda*norm(zeta).*V(:,2:end);
% % 
% % W_dot = - Gamma_w*( zeta*sigma');
% % W_dot(:,2:end)= W_dot(:,2:end) - Gamma_w*lambda*norm(zeta)*(W(:,2:end));
% % 
% % W_dot = W_dot';


%% Adaptation
W_update = W + T_sim*W_dot';
V_update = V + T_sim*V_dot;

%% re-compute v_ad

z = V*X_bar;
s=sigmoid(V*X_bar);

sigma = [1 ; s(:,1) ];
v_ad = W*sigma;

%% Compute v_ad_comp
Z = [ V,zeros(size(V,1),size(W,2));
    zeros(size(W,1),size(V,2)),W];
    
Z_norm = norm(Z,'fro');
Z_max = 2*min(size(W,1),size(W,2) )*min( size(V,1),size(V,2) );
Z_norm_unit = Z_norm;

K_r0= 0.02;
K_r1= 0;
v_r0 = -K_r0*zeta;
v_r1 = -K_r1*(Z_norm+Z_max)*zeta;

v_ad_comp = v_ad + v_r1 +v_r0;


end

== matlab function lib_controller/Controller/NDI+CA Controller/4DOF ANN+NDI+CA Controller - No massic update/On-line (adaptive) multi-layer NNs/Roll Channel/Roll 1HL NN/Roll NN ==
  data: X_bar input size=[12,1]; v_ad_comp output; e input; P input; B input; Roll_learnign_rate input size=1; Roll_reg_param input size=1; W input size=[1,31]; V input size=[30,12]; v_ad output; Z_norm_unit output; T_sim parameter; W_update output size=[1,31]; V_update output size=[30,12]
function [v_ad_comp,v_ad,Z_norm_unit,W_update,V_update]  = Roll_NN(X_bar,e,P,B,Roll_learnign_rate,Roll_reg_param,W,V,T_sim)

%% Compute prelimiary parametes
zeta= e'*P*B;
s=zeros(30,1);
z=s;
%% Feedforward
z = V*X_bar;
s=sigmoid(V*X_bar);

sigma = [1 ; s ];
% v_ad = W*sigma;

sigma_grad = (sigma.*(ones(size(sigma))-sigma));

%% Compute the gradients or adaptation laws
Gamma_w= Roll_learnign_rate; % W learnign rate
Gamma_v= Roll_learnign_rate; %V learning rate
lambda = Roll_reg_param;

V_dot=zeros(size(V));
W_dot=zeros(size(W'));

W_dot= -Gamma_w*(  (sigma - sigma_grad.*[1;z] ).*zeta  );
W_dot(2:end,1)= W_dot(2:end,1) - Gamma_w*lambda*norm(zeta)*(W(:,2:end))';

M = W'*zeta.*sigma_grad ;
V_dot= -Gamma_v*( M(2:end)*X_bar'  );
V_dot(:,2:end)= V_dot(:,2:end) - Gamma_v*lambda*norm(zeta).*V(:,2:end);


% Other way: Based on notes of Andrew NG
% % % W_dot=zeros(size(W));
% % % delta2=W'*zeta.*sigma_grad;
% % % 
% % % V_dot = - Gamma_v*( delta2(2:end)*X_bar');
% % % V_dot(:,2:end)= V_dot(:,2:end) - Gamma_v*lambda*norm(zeta).*V(:,2:end);
% % % 
% % % W_dot = - Gamma_w*( zeta*sigma');
% % % W_dot(:,2:end)= W_dot(:,2:end) - Gamma_w*lambda*norm(zeta)*(W(:,2:end));
% % % 
% % % W_dot = W_dot';


%% Adaptation
W_update = W + T_sim*W_dot';
V_update = V + T_sim*V_dot;

%% re-compute v_ad

s=sigmoid(V*X_bar);

sigma = [1 ; s(:,1) ];
v_ad = W*sigma;

%% Compute v_ad_comp
Z = [ V,zeros(size(V,1),size(W,2));
    zeros(size(W,1),size(V,2)),W];
    
Z_norm = norm(Z,'fro');
Z_max = 2*min(size(W,1),size(W,2) )*min( size(V,1),size(V,2) );
Z_norm_unit = Z_norm;

K_r0= 0;
K_r1= 0;
v_r0 = -K_r0*zeta;
v_r1 = -K_r1*(Z_norm+Z_max)*zeta;
v_ad_comp = v_ad + v_r1 +v_r0;

% % K_r1= 1;
% % v_r1 = - K_r1*(Z_norm+Z_max)*zeta;
% % 
% % v_ad_comp = v_ad + v_r1 ;



end

== matlab function lib_controller/Controller/NDI+CA Controller/4DOF ANN+NDI+CA Controller - No massic update/On-line (adaptive) multi-layer NNs/Roll Channel/Roll 2HL NN/Roll Multilayer NN ==
  data: X_bar input size=[12,1]; v_ad_comp output; e input size=1; P input; B input; Roll_learnign_rate input size=1; Roll_reg_param input size=1; Theta_1 input size=[30,12]; Theta_2 input size=[20,31]; Theta_3 input size=[1,21]; v_ad output; Z_norm_unit output; T_sim parameter; Theta_1_update output; Theta_2_update output; Theta_3_update output
function [v_ad_comp,v_ad,Z_norm_unit,Theta_1_update,Theta_2_update,Theta_3_update]  = Roll_ML_NN(X_bar,e,P,B,Roll_learnign_rate, Roll_reg_param,Theta_1,Theta_2,Theta_3,T_sim)

%% Compute prelimiary parameters
zeta= e'*P*B;

%% Feedforward. Layers: Sigmoidal, linear, linear

a2=[1 ;  sigmoid( Theta_1*X_bar )]; % Sigmoidal
a3=[1 ;  (Theta_2*a2)]; % Linear
% z4=Theta_3*a3;
% a4 = z4; % Linear
% v_ad =a4;

% Backward
% % delta4=zeta; % In this particular case of adaptive NN, this error is a weighted tracking error
delta3=Theta_3'*zeta;
delta2=Theta_2'*delta3(2:end).*(a2.*(ones(size(a2))-a2)); 


%% Compute the gradients or adaptation laws
Gamma_Theta_3= Roll_learnign_rate; %  learnign rate
Gamma_Theta_2 = Roll_learnign_rate; % learning rate
Gamma_Theta_1= Roll_learnign_rate; % learning rate
lambda = Roll_reg_param;    % Regularization constant

% % Theta_1_dot=zeros(size(Theta_1));
% % Theta_2_dot=zeros(size(Theta_2));
% % Theta_3_dot=zeros(size(Theta_3));

Theta_3_dot = -Gamma_Theta_3*zeta*a3' ;
Theta_3_dot(:,2:end) =  Theta_3_dot(:,2:end) - Gamma_Theta_3*lambda*norm(zeta).*Theta_3(:,2:end);

Theta_2_dot= -Gamma_Theta_2*( delta3(2:end)*a2'   + lambda*norm(zeta).*Theta_2);
Theta_2_dot(:,2:end) =  Theta_2_dot(:,2:end) - Gamma_Theta_2*lambda*norm(zeta).*Theta_2(:,2:end);

Theta_1_dot= -Gamma_Theta_1*( delta2(2:end)*X_bar'   + lambda*norm(zeta).*Theta_1);
Theta_1_dot(:,2:end) =  Theta_1_dot(:,2:end) - Gamma_Theta_1*lambda*norm(zeta).*Theta_1(:,2:end);


%% Adaptation
Theta_1_update = Theta_1 + T_sim*Theta_1_dot;
Theta_2_update = Theta_2 + T_sim*Theta_2_dot;
Theta_3_update = Theta_3 + T_sim*Theta_3_dot;

%% re-compute v_ad

a2=[1 ;  sigmoid( Theta_1_update*X_bar )]; % Sigmoidal
a3=[1 ;  (Theta_2_update*a2)]; % Linear
v_ad=Theta_3_update*a3;


%% Compute v_ad_comp
% Z = blkdiag( Theta_1_update , Theta_2_update , Theta_3_update );

Z =  [ Theta_1_update, zeros(size(Theta_1_update,1),size(Theta_2_update,2)) , zeros(size(Theta_1_update,1),size(Theta_3_update,2));
            zeros(size(Theta_2_update,1),size(Theta_1_update,2)) , Theta_2_update , zeros(size(Theta_2_update,1),size(Theta_3_update,2)) ;
            zeros(size(Theta_3_update,1),size(Theta_1_update,2)),zeros(size(Theta_3_update,1),size(Theta_2_update,2)),  Theta_3_update ];

Z_norm = norm(Z,'fro');
Z_max = min(size(Theta_1))*min(size(Theta_2))*min(size(Theta_3));
Z_norm_unit = Z_norm;

K_r0= 0.02;
K_r1= 0;
v_r0 = -K_r0*zeta;
v_r1 = -K_r1*(Z_norm+Z_max)*zeta;

v_ad_comp = v_ad + v_r1 +v_r0;


end

== matlab function lib_controller/Controller/NDI+CA Controller/4DOF ANN+NDI+CA Controller - No massic update/On-line (adaptive) multi-layer NNs/Yaw Channel/Yaw HL NN/Yaw NN ==
  data: X_bar input size=[12,1]; v_ad_comp output; e input; Ks input; B input; Long_learnign_rate input size=1; Long_reg_param input size=1; W input size=[1,31]; V input size=[30,12]; v_ad output; Z_norm_unit output; T_sim parameter; W_update output; V_update output
function [v_ad_comp,v_ad,Z_norm_unit,W_update,V_update]  = Yaw_NN(X_bar,e, Ks,B,Long_learnign_rate,Long_reg_param,W,V,T_sim)

%% Compute prelimiary parametes Ks(1)=K_b_alpha  and Ks(2) = K_b_q
P = [   1/Ks(1) , 1/(Ks(1)^2+Ks(1)*Ks(2));
     1/(Ks(1)^2+Ks(1)*Ks(2)) ,(Ks(1)^2+Ks(1)*Ks(2)+1)/(Ks(2)^2*Ks(1)+Ks(2)*Ks(1)^2) ];
zeta= e'*P*B;
s=zeros(30,1);
z=s;
%% Feedforward
z = V*X_bar;
s=sigmoid(V*X_bar);

sigma = [1 ; s ];
% v_ad = W*sigma;

sigma_grad = (sigma.*(ones(size(sigma))-sigma));

%% Compute the gradients or adaptation laws
Gamma_w= Long_learnign_rate; % W learnign rate
Gamma_v= Long_learnign_rate; %V learning rate
lambda = Long_reg_param;

V_dot=zeros(size(V));
W_dot=zeros(size(W'));

W_dot= -Gamma_w*(  (sigma - sigma_grad.*[1;z] ).*zeta  );
W_dot(2:end,1)= W_dot(2:end,1) - Gamma_w*lambda*norm(zeta)*(W(:,2:end))';

M = W'*zeta.*sigma_grad ;
V_dot= -Gamma_v*( M(2:end)*X_bar'  );
V_dot(:,2:end)= V_dot(:,2:end) - Gamma_v*lambda*norm(zeta).*V(:,2:end);


% % % Other way: Based on notes of Andrew NG
% % W_dot=zeros(size(W));
% % delta2=W'*zeta.*sigma_grad;
% % 
% % V_dot = - Gamma_v*( delta2(2:end)*X_bar');
% % V_dot(:,2:end)= V_dot(:,2:end) - Gamma_v*lambda*norm(zeta).*V(:,2:end);
% % 
% % W_dot = - Gamma_w*( zeta*sigma');
% % W_dot(:,2:end)= W_dot(:,2:end) - Gamma_w*lambda*norm(zeta)*(W(:,2:end));
% % 
% % W_dot = W_dot';


%% Adaptation
W_update = W + T_sim*W_dot';
V_update = V + T_sim*V_dot;

%% re-compute v_ad

z = V*X_bar;
s=sigmoid(V*X_bar);

sigma = [1 ; s(:,1) ];
v_ad = W*sigma;

%% Compute v_ad_comp
Z = [ V,zeros(size(V,1),size(W,2));
    zeros(size(W,1),size(V,2)),W];
    
Z_norm = norm(Z,'fro');
Z_max = 2*min(size(W,1),size(W,2) )*min( size(V,1),size(V,2) );
Z_norm_unit = Z_norm;

K_r0= 0.02;
K_r1= 0;
v_r0 = -K_r0*zeta;
v_r1 = -K_r1*(Z_norm+Z_max)*zeta;

v_ad_comp = v_ad + v_r1 +v_r0;


end

== matlab function lib_controller/Controller/NDI+CA Controller/4DOF ANN+NDI+CA Controller - No massic update/Adaptive NN/Crossed NN/MATLAB Function ==
  data: P1 input; P output; P2 input; P3 input; P4 input
function P = fcn(P1,P2,P3,P4)
%#codegen

P = blkdiag(P1,P2,P3,P4);

== matlab function lib_controller/Controller/NDI+CA Controller/4DOF ANN+NDI+CA Controller - No massic update/Adaptive NN/Crossed NN/MATLAB Function1 ==
  data: P1 input; P output; P2 input; P3 input; P4 input
function P = fcn(P1,P2,P3,P4)
%#codegen

P = blkdiag(P1,P2,P3,P4);

== matlab function lib_controller/Controller/NDI+CA Controller/4DOF ANN+NDI+CA Controller - No massic update/Adaptive NN/Crossed NN/MATLAB Function2 ==
  data: P1 input; P output; P2 input; P3 input; P4 input
function P = fcn(P1,P2,P3,P4)
%#codegen

P = [P1;P2;P3;P4];

== matlab function lib_controller/Controller/NDI+CA Controller/4DOF ANN+NDI+CA Controller - No massic update/Adaptive NN1/Complete crossed On-line (adaptive) multi-layer NN: AoA/Cross NN ==
  data: X_bar input size=[30,1]; v_ad_comp output size=4; e input size=6; P input size=[6,6]; B input size=[6,4]; learning_rate input size=1; Reg_param input size=1; W input size=[4,51]; V input size=[50,30]; v_ad output size=4; Z_norm_unit output size=1; T_sim parameter size=1; W_update output size=[4,51]; V_update output size=[50,30]
function [v_ad_comp,v_ad,Z_norm_unit,W_update,V_update]  = Cross_NN(X_bar,e, P, B,learning_rate,Reg_param,W,V,T_sim)

%% Compute prelimiary parameters 
zeta= e'*P*B;

%% Feedforward
z = V*X_bar;
s=sigmoid(V*X_bar);

sigma = [1 ; s ];
% v_ad = W*sigma;

sigma_grad = (sigma.*(ones(size(sigma))-sigma));

%% Compute the gradients or adaptation laws
Gamma_w= learning_rate; % W learnign rate
Gamma_v= learning_rate; %V learning rate
lambda = Reg_param;

V_dot=zeros(size(V));
W_dot=zeros(size(W));

W_dot= -Gamma_w*(  (sigma - sigma_grad.*[1;z] )*zeta  )';
W_dot(:,2:end)= W_dot(:,2:end) - Gamma_w*lambda*norm(zeta)*(W(:,2:end));

M = W'*zeta'.*sigma_grad ;
V_dot= -Gamma_v*( M(2:end)*X_bar'  );
V_dot(:,2:end)= V_dot(:,2:end) - Gamma_v*lambda*norm(zeta).*V(:,2:end);

% % % % Other way: Based on notes of Andrew NG
% % % 
% % % delta2=W'*zeta'.*sigma_grad;
% % % 
% % % V_dot = - Gamma_v*( delta2(2:end)*X_bar');
% % % V_dot(:,2:end)= V_dot(:,2:end) - Gamma_v*lambda*norm(zeta).*V(:,2:end);
% % % 
% % % W_dot = - Gamma_w*( sigma*zeta)';
% % % W_dot(:,2:end)= W_dot(:,2:end) - Gamma_w*lambda*norm(zeta)*(W(:,2:end));

%% Adaptation
W_update = W + T_sim*W_dot;
V_update = V + T_sim*V_dot;

%% Re-compute v_ad
s=sigmoid(V_update*X_bar);

sigma = [1 ; s(:,1) ];
v_ad = W_update*sigma;

%% Compute v_ad_comp (add robustifying terms)
Z = [ V,zeros(size(V,1),size(W,2));
    zeros(size(W,1),size(V,2)),W];
    
Z_norm = norm(Z,'fro');
Z_max = 2*min(size(W,1),size(W,2) )*min(size(V,1),size(V,2));
Z_norm_unit = Z_norm;

K_r0= 0.02;
K_r1= 0;
v_r0 = -K_r0*zeta';
v_r1 = -K_r1*(Z_norm+Z_max)*zeta';

v_ad_comp = v_ad + v_r1 +v_r0;
end

== matlab function lib_controller/Controller/NDI+CA Controller/4DOF ANN+NDI+CA Controller - No massic update/Adaptive NN1/Complete crossed On-line (adaptive) multi-layer NN: AoA/MATLAB Function ==
  data: P1 input; P output; P2 input; P3 input; P4 input
function P = fcn(P1,P2,P3,P4)
%#codegen

P = blkdiag(P1,P2,P3,P4);

== matlab function lib_controller/Controller/NDI+CA Controller/4DOF ANN+NDI+CA Controller - No massic update/Adaptive NN1/Complete crossed On-line (adaptive) multi-layer NN: AoA/MATLAB Function1 ==
  data: P1 input; P output; P2 input; P3 input; P4 input
function P = fcn(P1,P2,P3,P4)
%#codegen

P = blkdiag(P1,P2,P3,P4);

== matlab function lib_controller/Controller/NDI+CA Controller/4DOF ANN+NDI+CA Controller - No massic update/Adaptive NN1/Complete crossed On-line (adaptive) multi-layer NN: AoA/MATLAB Function2 ==
  data: P1 input; P output; P2 input; P3 input; P4 input
function P = fcn(P1,P2,P3,P4)
%#codegen

P = [P1;P2;P3;P4];

== matlab function lib_controller/Controller/NDI+CA Controller/4DOF NDI+CA Controller - No massic update/F(X)1 ==
  data: fx output size=[4,1]; prev_input input size=[9,1]; gforce_body input size=[3,1]; omega_body input size=[3,1]; v_body input size=[3,1]
function fx = fx(prev_input, gforce_body, omega_body, v_body)
    % Calculates f_hat(x). The expression is calculated in NDI_components
    % x_dot = f(x) + g(x,u)
    %   g(x,u) ~= g(x,u0) + jac(g(x,u), u)(u0) * (u - u0)
    %   g(x,u) ~= h(x,u0) + jac(g(x,u), u)(u0) * u
    % x_dot = f_hat(x) + jac(g(x,u), u) * u
    %   f_hat(x) = f(x) + g(x,u0) - jac(g(x,u), u)(u0) *  u0
    %   g_hat(x) = jac(g(x,u), u)(u0)
    % x_dot = f_hat(x) + g_hat(x) * u
    tau1_0 = prev_input(1);
    eta1_0 = prev_input(2);
    gamma1_0 = prev_input(3);
    tau2_0 = prev_input(4);
    eta2_0 = prev_input(5);
    gamma2_0 = prev_input(6);
    tau3_0 = prev_input(7);
    eta3_0 = prev_input(8);
    gamma3_0 = prev_input(9);
    Gx =  gforce_body(1);
    Gy =  gforce_body(2);
    Gz =  gforce_body(3);
    U = v_body(1);
    V = v_body(2);
    W = v_body(3);
    P = omega_body(1);
    Q = omega_body(2);
    R = omega_body(3);

    % This matrix was precomputed in NDI_components.m
    % TODO Precompute sines and cosines to improve performance. Some
    % repeated terms can also be precomputed
    
 % Kt = 29.6 Kq = 0.3
 fx = [... 
                    - 0.0015*P^2 - 1.0*V*P - 0.0015*Q^2 + U*Q + 0.2849*Gz - 7.379*eta1_0*tau1_0*sin(eta1_0);
              1.541*eta1_0*tau1_0*cos(eta1_0) - 0.8756*Q*R - 0.0436*P*Q + 0.04359*eta1_0*tau1_0*sin(eta1_0);
 0.03918*P^2 + 0.9007*P*R - 0.03918*R^2 - 1.469*eta1_0*tau1_0*cos(eta1_0) + 43.76*eta1_0*tau1_0*sin(eta1_0);
                0.0436*Q*R - 0.1269*P*Q - 26.0*eta1_0*tau1_0*cos(eta1_0) - 0.8729*eta1_0*tau1_0*sin(eta1_0)];    
 
% Kt = 15 Kq = 0.07
%                          - 0.0015*P^2 - 1.0*V*P - 0.0015*Q^2 + 1.0*U*Q + 0.2849*Gz - 4.2735*eta1_0*tau1_0*sin(eta1_0);
%                   0.89255*eta1_0*tau1_0*cos(eta1_0) - 0.87555*Q*R - 0.043605*P*Q + 0.010171*eta1_0*tau1_0*sin(eta1_0);
%      0.039179*P^2 + 0.90066*P*R - 0.039179*R^2 - 0.34281*eta1_0*tau1_0*cos(eta1_0) + 25.344*eta1_0*tau1_0*sin(eta1_0);
%                      0.043605*Q*R - 0.12686*P*Q - 15.06*eta1_0*tau1_0*cos(eta1_0) - 0.20367*eta1_0*tau1_0*sin(eta1_0)];

== matlab function lib_controller/Controller/NDI+CA Controller/4DOF NDI+CA Controller - No massic update/G(X) 4DOF_WPQR1 ==
  data: gx output size=[4,4]; prev_input input size=[9,1]
function gx = gx(prev_input)
    % Calculates f_hat(x). The expression is calculated in NDI_components
    % x_dot = f(x) + g(x,u)
    %   g(x,u) ~= g(x,u0) + jac(g(x,u), u)(u0) * (u - u0)
    %   g(x,u) ~= h(x,u0) + jac(g(x,u), u)(u0) * u
    % x_dot = f_hat(x) + jac(g(x,u), u) * u
    %   f_hat(x) = f(x) + g(x,u0) - jac(g(x,u), u)(u0) *  u0
    %   g_hat(x) = jac(g(x,u), u)(u0)
    % x_dot = f_hat(x) + g_hat(x) * u
    tau1_0 = prev_input(1);
    eta1_0 = prev_input(2);
    gamma1_0 = prev_input(3);
    tau2_0 = prev_input(4);
    eta2_0 = prev_input(5);
    gamma2_0 = prev_input(6);
    tau3_0 = prev_input(7);
    eta3_0 = prev_input(8);
    gamma3_0 = prev_input(9);
    
    % This matrix was precomputed in NDI_components.m
    % TODO Precompute sines and cosines to improve performance. Some
    % repeated terms can also be precomputed
    
    % Kt = 29.6 Kq = 0.3
    gx = [...
                          -7.379*cos(eta1_0),                                7.379*tau1_0*sin(eta1_0), -7.379,  -7.379;
     0.04359*cos(eta1_0) - 1.541*sin(eta1_0), - 1.541*tau1_0*cos(eta1_0) - 0.04359*tau1_0*sin(eta1_0), -48.41,   48.32;
       43.76*cos(eta1_0) + 1.469*sin(eta1_0),     1.469*tau1_0*cos(eta1_0) - 43.76*tau1_0*sin(eta1_0), -21.88,  -21.88;
       26.0*sin(eta1_0) - 0.8729*cos(eta1_0),     26.0*tau1_0*cos(eta1_0) + 0.8729*tau1_0*sin(eta1_0),  1.997, -0.2515];
 
% Kt = 15 Kq = 0.07
%                        -4.274*cos(eta1_0),                                 4.274*tau1_0*sin(eta1_0), -4.274,  -4.274;
%  0.01017*cos(eta1_0) - 0.8926*sin(eta1_0), - 0.8926*tau1_0*cos(eta1_0) - 0.01017*tau1_0*sin(eta1_0), -28.02,    28.0;
%    25.34*cos(eta1_0) + 0.3428*sin(eta1_0),     0.3428*tau1_0*cos(eta1_0) - 25.34*tau1_0*sin(eta1_0), -12.67,  -12.67;
%    15.06*sin(eta1_0) - 0.2037*cos(eta1_0),     15.06*tau1_0*cos(eta1_0) + 0.2037*tau1_0*sin(eta1_0), 0.8549, -0.4475];

== matlab function lib_controller/Controller/NDI+CA Controller/4DOF NDI+CA Controller - No massic update/Rotational Kinematics ==
  data: PQR output; Eulerdot input; Euler input
function PQR = rot_kin(Eulerdot,Euler)
%solves rotational kinematic equations
Phi = Euler(1);
Theta = Euler(2);
Psi = Euler(3);
A = [1 sin(Phi)*tan(Theta) cos(Phi)*tan(Theta);
     0 cos(Phi) -sin(Phi);
     0 sin(Phi)*sec(Theta) cos(Phi)*sec(Theta)];
PQR = A'*Eulerdot;
end

== matlab function lib_controller/Controller/NDI+CA Controller/9DOF ANN+NDI+CA Controller - No massic update/Adaptive NN/Crossed NN/Cross NN ==
  data: X_bar input size=[38,1]; v_ad_comp output size=6; e input size=8; P input size=[8,8]; B input size=[8,6]; learning_rate input size=1; Reg_param input size=2; W input size=[6,51]; V input size=[50,38]; v_ad output size=6; Z_norm_unit output size=1; T_sim parameter size=1; W_update output size=[6,51]; V_update output size=[50,38]
function [v_ad_comp,v_ad,Z_norm_unit,W_update,V_update]  = Cross_NN(X_bar,e, P, B,learning_rate,Reg_param,W,V,T_sim)

%% Compute prelimiary parameters 
zeta= e'*P*B;

%% Feedforward
z = V*X_bar;
s=sigmoid(V*X_bar);

sigma = [1 ; s ];
% v_ad = W*sigma;

sigma_grad = (sigma.*(ones(size(sigma))-sigma));

%% Compute the gradients or adaptation laws
Gamma_w= learning_rate; % W learnign rate
Gamma_v= learning_rate; %V learning rate
lambda_v = Reg_param(1);
lambda_w = Reg_param(2);

V_dot=zeros(size(V));
W_dot=zeros(size(W));

W_dot= -Gamma_w*(  (sigma - sigma_grad.*[1;z] )*zeta  )';
W_dot(:,2:end)= W_dot(:,2:end) - Gamma_w*lambda_w*norm(zeta)*(W(:,2:end));

M = W'*zeta'.*sigma_grad ;
V_dot= -Gamma_v*( M(2:end)*X_bar'  );
V_dot(:,2:end)= V_dot(:,2:end) - Gamma_v*lambda_v*norm(zeta).*V(:,2:end);

% % % % Other way: Based on notes of Andrew NG
% % % 
% % % delta2=W'*zeta'.*sigma_grad;
% % % 
% % % V_dot = - Gamma_v*( delta2(2:end)*X_bar');
% % % V_dot(:,2:end)= V_dot(:,2:end) - Gamma_v*lambda*norm(zeta).*V(:,2:end);
% % % 
% % % W_dot = - Gamma_w*( sigma*zeta)';
% % % W_dot(:,2:end)= W_dot(:,2:end) - Gamma_w*lambda*norm(zeta)*(W(:,2:end));

%% Adaptation scalled with loop time
W_update = W + T_sim*W_dot;
V_update = V + T_sim*V_dot;

%% Re-compute v_ad
s=sigmoid(V_update*X_bar);

sigma = [1 ; s(:,1) ];
v_ad = W_update*sigma;

%% Compute v_ad_comp (add robustifying terms)
Z = [ V,zeros(size(V,1),size(W,2));
    zeros(size(W,1),size(V,2)),W];
    
Z_norm = norm(Z,'fro');
% Z_max = 2*min(size(W,1),size(W,2) )*min(size(V,1),size(V,2));
Z_max = 1;
Z_norm_unit = Z_norm;

% K_r0= 0.02;
% K_r1= 0;
K_r0= 1;
K_r1= 1;

v_r0 = -K_r0*zeta';
v_r1 = -K_r1*(Z_norm+Z_max)*zeta';

v_ad_comp = v_ad + v_r1 +v_r0;
end

== matlab function lib_controller/Controller/NDI+CA Controller/9DOF ANN+NDI+CA Controller - No massic update/Adaptive NN/Crossed NN/MATLAB Function2 ==
  data: P1 input; P output; P2 input; P3 input; P4 input; P5 input; P6 input
function P = fcn(P1,P2,P3,P4,P5,P6)
%#codegen

P = blkdiag(P1,P2,P3,P4,P5,P6);

== matlab function lib_controller/Controller/NDI+CA Controller/9DOF ANN+NDI+CA Controller - No massic update/Adaptive NN/Crossed NN/MATLAB Function1 ==
  data: P1 input; P output; P2 input; P3 input; P4 input; P5 input; P6 input
function P = fcn(P1,P2,P3,P4,P5,P6)
%#codegen

P = blkdiag(P1,P2,P3,P4,P5,P6);

== matlab function lib_controller/Controller/NDI+CA Controller/9DOF ANN+NDI+CA Controller - No massic update/Adaptive NN/Crossed NN/MATLAB Function3 ==
  data: P1 input; P output size=8; P2 input; P3 input; P4 input; P5 input; P6 input
function P = fcn(P1,P2,P3,P4,P5,P6)
%#codegen

P = [P1;P2;P3;P4;P5;P6];
